simulink model "Constant_TestGen27"  (R2017b)
settings: Solver=FixedStepDiscrete  StartTime=0.0  StopTime=10.0  RelTol=1e-3
undefined symbols (not defined in the file): Block_TestLib, enable
settings Model: Creator=ktrinh  LastModifiedBy=ktrinh
settings DebuggingCC: ParameterOverflowMsg=none

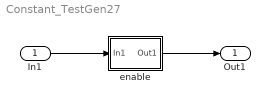
== system Constant_TestGen27 ==
  In1 : Inport
  enable : Subsystem  AncestorBlock=Block_TestLib/enable
  Out1 : Outport
  wires:
  In1/1 -> enable/1(In1)
  enable/1(Out1) -> Out1/1

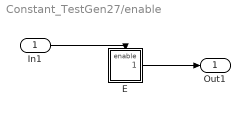
== system Constant_TestGen27/enable ==
  In1 : Inport  OutDataTypeStr=boolean
  E : Subsystem  TreatAsAtomicUnit=on
  Out1 : Outport
  wires:
  In1/1 -> E/Enable
  E/1(Out1) -> Out1/1

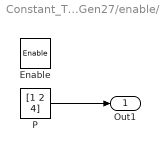
== system Constant_TestGen27/enable/E ==
  Enable : EnablePort
  P : Constant  Value=[1 2 4]  VectorParams1D=off  OutDataTypeStr=single
  Out1 : Outport
  wires:
  P/1 -> Out1/1
